simulink model "empirical_cell_twaice_balancing"  (R2024b)
settings: Solver=FixedStepAuto  StartTime=0.0  StopTime=inf  FixedStep=1  RelTol=1e-3
values from neighbouring files (symbols this model uses):
  act = 1    [RunMe_TWAICE_Cell_Model_Farasis_P75_75Ah_v8_1_3.m]
  lic_no = fin_convert(Prod_lic)    [RunMe_TWAICE_Cell_Model_Farasis_P75_75Ah_v8_1_3.m]
  Ts = 1    [RunMe_TWAICE_Cell_Model_Farasis_P75_75Ah_v8_1_3.m]
undefined symbols (not defined in the file or in its folder): DWORK0, DWORK1, DWORK10, DWORK11, DWORK12, DWORK13, DWORK14, DWORK15, DWORK16, DWORK17, DWORK18, DWORK19, DWORK2, DWORK20, DWORK22, DWORK23, DWORK24, DWORK25, DWORK26, DWORK27, DWORK28, DWORK29, DWORK3, DWORK30, DWORK31, DWORK32, DWORK33, DWORK34, DWORK35, DWORK36, DWORK4, DWORK5, DWORK6, DWORK7, DWORK8, DWORK9, SOHc_init, SOHr_init
libraries: fl_lib x73, nesl_utility x32, ee_lib x8
(part 2 of 4)

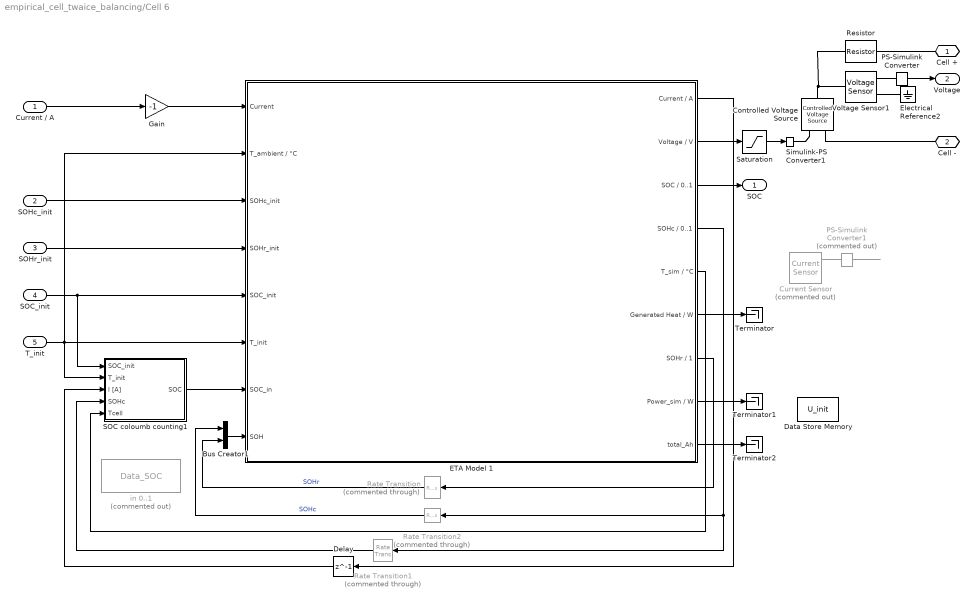
== system empirical_cell_twaice_balancing/Cell 6 ==
  "Current / A " : Inport  OutDataTypeStr=double  PortDimensions=1
  SOHc_init : Inport  Port=2
  SOHr_init : Inport  Port=3
  SOC_init : Inport  Port=4
  T_init : Inport  Port=5
  Bus Creator1 : BusCreator  Inputs=2
  Controlled Voltage Source : fl_lib/Electrical/Electrical Sources/Controlled Voltage Source
  Current Sensor : fl_lib/Electrical/Electrical Sensors/Current Sensor  Commented=on
  Data Store Memory : DataStoreMemory  DataStoreName=U_init  WriteAfterWriteMsg=warning  ShowAdditionalParam=off
  Delay : Delay  DelayLength=1
  ETA Model 1 : Subsystem  mask{sfcnParam1=Ts, sfcnParam2=act, sfcnParam3=lic_no}
      mask prompts: sfcnParam1 "Ts:"; sfcnParam2 "act:"; sfcnParam3 "lic_no:"
      mask help: Simulink:masks:GenSFuncDesc_MD
      mask Help: eval('feval(''rtwprivate'',''rtwhelpview'',''rtw_sfcn_block'')');
  Electrical Reference2 : fl_lib/Electrical/Electrical Elements/Electrical Reference
  Gain : Gain  Gain=-1
  PS-Simulink Converter : nesl_utility/PS-Simulink Converter  PhysicalDomain=network_engine_domain  SubClassName=ps_output  LeftPortType=input  RightPortType=output  PseudoPeriodic=off  Frequencies=[]  VectorFormat=inherit  Unit=inherit  AffineConversion=on
  PS-Simulink Converter1 : nesl_utility/PS-Simulink Converter  Commented=on  PhysicalDomain=network_engine_domain  SubClassName=ps_output  LeftPortType=input  RightPortType=output  PseudoPeriodic=off  Frequencies=[]  VectorFormat=inherit  Unit=inherit  AffineConversion=on
  Rate Transition : RateTransition  Commented=through  InitialCondition=SOHr_init
  Rate Transition1 : RateTransition  Commented=through  InitialCondition=SOHc_init
  Rate Transition2 : RateTransition  Commented=through  InitialCondition=SOHc_init
  Resistor : fl_lib/Electrical/Electrical Elements/Resistor  R=1 mOhm  i_specify=off  i_priority=None  i=0 A  i_nominal_specify=off  i_nominal_value=1  i_nominal_unit=A  v_specify=off  v_priority=None  v=0 V  v_nominal_specify=off  v_nominal_value=1  v_nominal_unit=V
  SOC coloumb counting1 : Subsystem  mask{sfcnParam1=Ts}
      mask prompts: sfcnParam1 "Ts:"
      mask help: Simulink:masks:GenSFuncDesc_MD
      mask Help: eval('feval(''rtwprivate'',''rtwhelpview'',''rtw_sfcn_block'')');
  Saturation : Saturate  UpperLimit=4.15  LowerLimit=2.8
  Simulink-PS Converter1 : nesl_utility/Simulink-PS Converter  PhysicalDomain=network_engine_domain  SubClassName=ps_input  LeftPortType=input  RightPortType=output  PseudoPeriodic=off  Frequencies=[]  NoiseDistribution=none  NoiseParameters=[]  Unit=1  AffineConversion=on  FilteringAndDerivatives=provide  SimscapeFilterOrder=1  InputFilterTimeConstant=0.001  UdotUserProvided=0
  Terminator : Terminator
  Terminator1 : Terminator
  Terminator2 : Terminator
  Voltage Sensor1 : fl_lib/Electrical/Electrical Sensors/Voltage Sensor
  in 0..1 : FromWorkspace  Commented=on  VariableName=Data_SOC  SampleTime=Ts  OutputAfterFinalValue=Setting to zero
  Cell + : PMIOPort  Side=Right
  Cell - : PMIOPort  Port=2  Side=Right
  SOC : Outport
  Voltage : Outport  Port=2
  wires:
  Rate Transition/1 -> Bus Creator1/2  "SOHr"
  T_init/1 -> ETA Model 1/2(T_ambient / °C), SOC coloumb counting1/2(T_init), ETA Model 1/6(T_init)
  ETA Model 1/4(SOHc / 0..1) -> Rate Transition2/1, Rate Transition1/1
  SOC_init/1 -> SOC coloumb counting1/1(SOC_init), ETA Model 1/5(SOC_init)
  Rate Transition1/1 -> SOC coloumb counting1/4(SOHc)
  SOHc_init/1 -> ETA Model 1/3(SOHc_init)
  ETA Model 1/9(total_Ah) -> Terminator2/1
  ETA Model 1/7(SOHr / 1) -> Rate Transition/1
  ETA Model 1/1(Current / A) -> Delay/1
  ETA Model 1/5(T_sim / °C) -> SOC coloumb counting1/5(Tcell)
  SOC coloumb counting1/1(SOC) -> ETA Model 1/7(SOC_in)
  ETA Model 1/8(Power_sim / W) -> Terminator1/1
  Delay/1 -> SOC coloumb counting1/3(I [A])
  Bus Creator1/1 -> ETA Model 1/8(SOH)
  Rate Transition2/1 -> Bus Creator1/1  "SOHc"
  "Current / A "/1 -> Gain/1
  SOHr_init/1 -> ETA Model 1/4(SOHr_init)
  ETA Model 1/6(Generated Heat / W) -> Terminator/1
  Gain/1 -> ETA Model 1/1("Current ")
  ETA Model 1/3(SOC / 0..1) -> SOC/1
  PS-Simulink Converter/1 -> Voltage/1
  ETA Model 1/2(Voltage / V) -> Saturation/1
  PS-Simulink Converter1/1 -> ?
  Saturation/1 -> Simulink-PS Converter1/1
  connections:
  Cell +/RConn1 -- Resistor/RConn1
  Electrical Reference2/LConn1 -- Voltage Sensor1/RConn2
  PS-Simulink Converter/LConn1 -- Voltage Sensor1/RConn1
  Current Sensor/RConn1 -- PS-Simulink Converter1/LConn1
  Controlled Voltage Source/RConn2 -- Cell -/RConn1
  Simulink-PS Converter1/RConn1 -- Controlled Voltage Source/RConn1
  Voltage Sensor1/LConn1 -- Resistor/LConn1 -- Controlled Voltage Source/LConn1

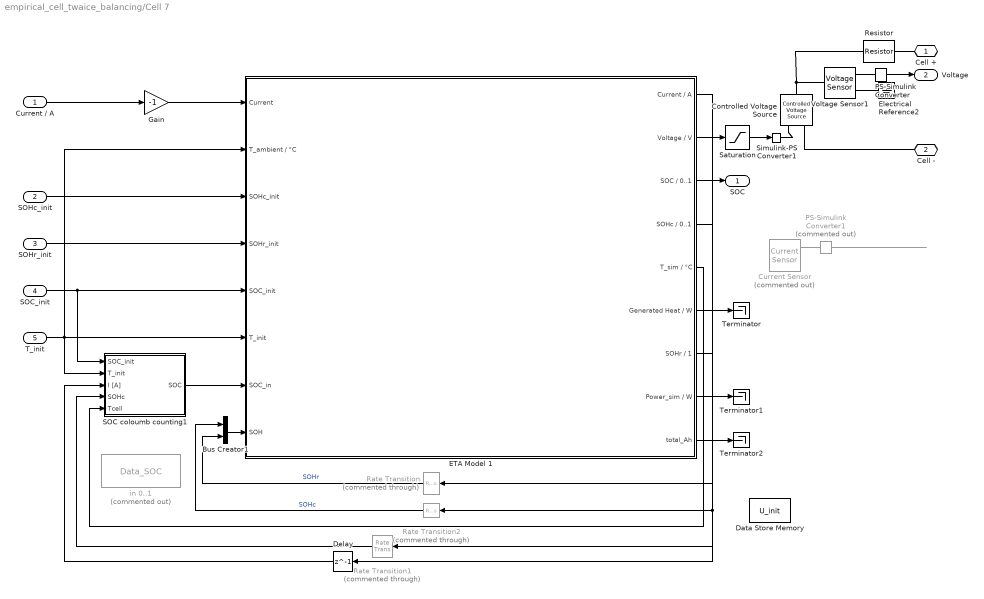
== system empirical_cell_twaice_balancing/Cell 7 ==
  "Current / A " : Inport  OutDataTypeStr=double  PortDimensions=1
  SOHc_init : Inport  Port=2
  SOHr_init : Inport  Port=3
  SOC_init : Inport  Port=4
  T_init : Inport  Port=5
  Bus Creator1 : BusCreator  Inputs=2
  Controlled Voltage Source : fl_lib/Electrical/Electrical Sources/Controlled Voltage Source
  Current Sensor : fl_lib/Electrical/Electrical Sensors/Current Sensor  Commented=on
  Data Store Memory : DataStoreMemory  DataStoreName=U_init  WriteAfterWriteMsg=warning  ShowAdditionalParam=off
  Delay : Delay  DelayLength=1
  ETA Model 1 : Subsystem  mask{sfcnParam1=Ts, sfcnParam2=act, sfcnParam3=lic_no}
      mask prompts: sfcnParam1 "Ts:"; sfcnParam2 "act:"; sfcnParam3 "lic_no:"
      mask help: Simulink:masks:GenSFuncDesc_MD
      mask Help: eval('feval(''rtwprivate'',''rtwhelpview'',''rtw_sfcn_block'')');
  Electrical Reference2 : fl_lib/Electrical/Electrical Elements/Electrical Reference
  Gain : Gain  Gain=-1
  PS-Simulink Converter : nesl_utility/PS-Simulink Converter  PhysicalDomain=network_engine_domain  SubClassName=ps_output  LeftPortType=input  RightPortType=output  PseudoPeriodic=off  Frequencies=[]  VectorFormat=inherit  Unit=inherit  AffineConversion=on
  PS-Simulink Converter1 : nesl_utility/PS-Simulink Converter  Commented=on  PhysicalDomain=network_engine_domain  SubClassName=ps_output  LeftPortType=input  RightPortType=output  PseudoPeriodic=off  Frequencies=[]  VectorFormat=inherit  Unit=inherit  AffineConversion=on
  Rate Transition : RateTransition  Commented=through  InitialCondition=SOHr_init
  Rate Transition1 : RateTransition  Commented=through  InitialCondition=SOHc_init
  Rate Transition2 : RateTransition  Commented=through  InitialCondition=SOHc_init
  Resistor : fl_lib/Electrical/Electrical Elements/Resistor  R=1 mOhm  i_specify=off  i_priority=None  i=0 A  i_nominal_specify=off  i_nominal_value=1  i_nominal_unit=A  v_specify=off  v_priority=None  v=0 V  v_nominal_specify=off  v_nominal_value=1  v_nominal_unit=V
  SOC coloumb counting1 : Subsystem  mask{sfcnParam1=Ts}
      mask prompts: sfcnParam1 "Ts:"
      mask help: Simulink:masks:GenSFuncDesc_MD
      mask Help: eval('feval(''rtwprivate'',''rtwhelpview'',''rtw_sfcn_block'')');
  Saturation : Saturate  UpperLimit=4.15  LowerLimit=2.8
  Simulink-PS Converter1 : nesl_utility/Simulink-PS Converter  PhysicalDomain=network_engine_domain  SubClassName=ps_input  LeftPortType=input  RightPortType=output  PseudoPeriodic=off  Frequencies=[]  NoiseDistribution=none  NoiseParameters=[]  Unit=1  AffineConversion=on  FilteringAndDerivatives=provide  SimscapeFilterOrder=1  InputFilterTimeConstant=0.001  UdotUserProvided=0
  Terminator : Terminator
  Terminator1 : Terminator
  Terminator2 : Terminator
  Voltage Sensor1 : fl_lib/Electrical/Electrical Sensors/Voltage Sensor
  in 0..1 : FromWorkspace  Commented=on  VariableName=Data_SOC  SampleTime=Ts  OutputAfterFinalValue=Setting to zero
  Cell + : PMIOPort  Side=Right
  Cell - : PMIOPort  Port=2  Side=Right
  SOC : Outport
  Voltage : Outport  Port=2
  wires:
  Rate Transition/1 -> Bus Creator1/2  "SOHr"
  T_init/1 -> ETA Model 1/2(T_ambient / °C), SOC coloumb counting1/2(T_init), ETA Model 1/6(T_init)
  ETA Model 1/4(SOHc / 0..1) -> Rate Transition2/1, Rate Transition1/1
  SOC_init/1 -> SOC coloumb counting1/1(SOC_init), ETA Model 1/5(SOC_init)
  Rate Transition1/1 -> SOC coloumb counting1/4(SOHc)
  SOHc_init/1 -> ETA Model 1/3(SOHc_init)
  ETA Model 1/7(SOHr / 1) -> Rate Transition/1
  ETA Model 1/1(Current / A) -> Delay/1
  ETA Model 1/5(T_sim / °C) -> SOC coloumb counting1/5(Tcell)
  SOC coloumb counting1/1(SOC) -> ETA Model 1/7(SOC_in)
  Delay/1 -> SOC coloumb counting1/3(I [A])
  Bus Creator1/1 -> ETA Model 1/8(SOH)
  Rate Transition2/1 -> Bus Creator1/1  "SOHc"
  SOHr_init/1 -> ETA Model 1/4(SOHr_init)
  ETA Model 1/6(Generated Heat / W) -> Terminator/1
  Gain/1 -> ETA Model 1/1("Current ")
  ETA Model 1/8(Power_sim / W) -> Terminator1/1
  ETA Model 1/3(SOC / 0..1) -> SOC/1
  PS-Simulink Converter/1 -> Voltage/1
  "Current / A "/1 -> Gain/1
  ETA Model 1/2(Voltage / V) -> Saturation/1
  ETA Model 1/9(total_Ah) -> Terminator2/1
  PS-Simulink Converter1/1 -> ?
  Saturation/1 -> Simulink-PS Converter1/1
  connections:
  PS-Simulink Converter/LConn1 -- Voltage Sensor1/RConn1
  Simulink-PS Converter1/RConn1 -- Controlled Voltage Source/RConn1
  Voltage Sensor1/LConn1 -- Resistor/LConn1 -- Controlled Voltage Source/LConn1
  Controlled Voltage Source/RConn2 -- Cell -/RConn1
  Electrical Reference2/LConn1 -- Voltage Sensor1/RConn2
  Current Sensor/RConn1 -- PS-Simulink Converter1/LConn1
  Cell +/RConn1 -- Resistor/RConn1

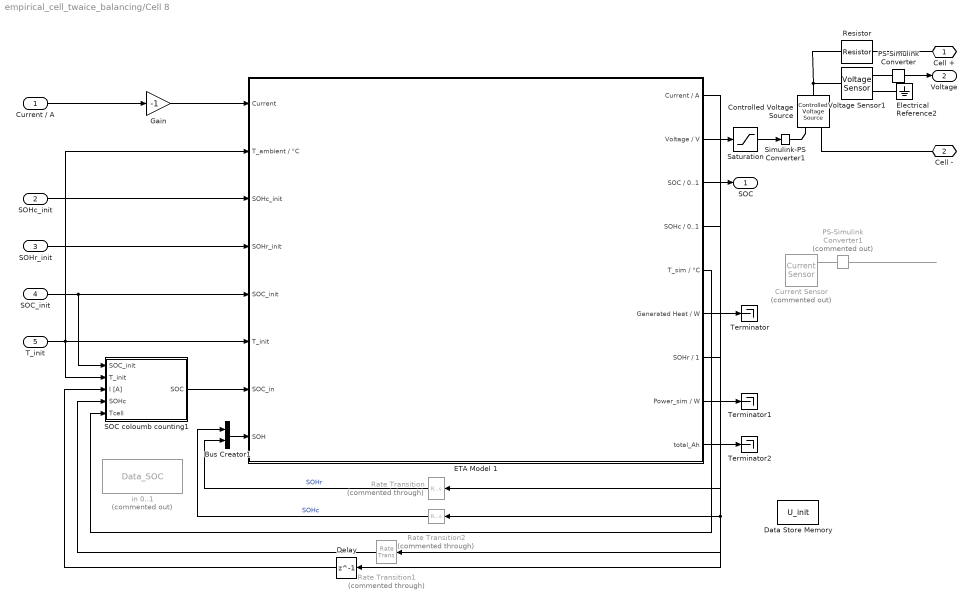
== system empirical_cell_twaice_balancing/Cell 8 ==
  "Current / A " : Inport  OutDataTypeStr=double  PortDimensions=1
  SOHc_init : Inport  Port=2
  SOHr_init : Inport  Port=3
  SOC_init : Inport  Port=4
  T_init : Inport  Port=5
  Bus Creator1 : BusCreator  Inputs=2
  Controlled Voltage Source : fl_lib/Electrical/Electrical Sources/Controlled Voltage Source
  Current Sensor : fl_lib/Electrical/Electrical Sensors/Current Sensor  Commented=on
  Data Store Memory : DataStoreMemory  DataStoreName=U_init  WriteAfterWriteMsg=warning  ShowAdditionalParam=off
  Delay : Delay  DelayLength=1
  ETA Model 1 : Subsystem  mask{sfcnParam1=Ts, sfcnParam2=act, sfcnParam3=lic_no}
      mask prompts: sfcnParam1 "Ts:"; sfcnParam2 "act:"; sfcnParam3 "lic_no:"
      mask help: Simulink:masks:GenSFuncDesc_MD
      mask Help: eval('feval(''rtwprivate'',''rtwhelpview'',''rtw_sfcn_block'')');
  Electrical Reference2 : fl_lib/Electrical/Electrical Elements/Electrical Reference
  Gain : Gain  Gain=-1
  PS-Simulink Converter : nesl_utility/PS-Simulink Converter  PhysicalDomain=network_engine_domain  SubClassName=ps_output  LeftPortType=input  RightPortType=output  PseudoPeriodic=off  Frequencies=[]  VectorFormat=inherit  Unit=inherit  AffineConversion=on
  PS-Simulink Converter1 : nesl_utility/PS-Simulink Converter  Commented=on  PhysicalDomain=network_engine_domain  SubClassName=ps_output  LeftPortType=input  RightPortType=output  PseudoPeriodic=off  Frequencies=[]  VectorFormat=inherit  Unit=inherit  AffineConversion=on
  Rate Transition : RateTransition  Commented=through  InitialCondition=SOHr_init
  Rate Transition1 : RateTransition  Commented=through  InitialCondition=SOHc_init
  Rate Transition2 : RateTransition  Commented=through  InitialCondition=SOHc_init
  Resistor : fl_lib/Electrical/Electrical Elements/Resistor  R=1 mOhm  i_specify=off  i_priority=None  i=0 A  i_nominal_specify=off  i_nominal_value=1  i_nominal_unit=A  v_specify=off  v_priority=None  v=0 V  v_nominal_specify=off  v_nominal_value=1  v_nominal_unit=V
  SOC coloumb counting1 : Subsystem  mask{sfcnParam1=Ts}
      mask prompts: sfcnParam1 "Ts:"
      mask help: Simulink:masks:GenSFuncDesc_MD
      mask Help: eval('feval(''rtwprivate'',''rtwhelpview'',''rtw_sfcn_block'')');
  Saturation : Saturate  UpperLimit=4.15  LowerLimit=2.8
  Simulink-PS Converter1 : nesl_utility/Simulink-PS Converter  PhysicalDomain=network_engine_domain  SubClassName=ps_input  LeftPortType=input  RightPortType=output  PseudoPeriodic=off  Frequencies=[]  NoiseDistribution=none  NoiseParameters=[]  Unit=1  AffineConversion=on  FilteringAndDerivatives=provide  SimscapeFilterOrder=1  InputFilterTimeConstant=0.001  UdotUserProvided=0
  Terminator : Terminator
  Terminator1 : Terminator
  Terminator2 : Terminator
  Voltage Sensor1 : fl_lib/Electrical/Electrical Sensors/Voltage Sensor
  in 0..1 : FromWorkspace  Commented=on  VariableName=Data_SOC  SampleTime=Ts  OutputAfterFinalValue=Setting to zero
  Cell + : PMIOPort  Side=Right
  Cell - : PMIOPort  Port=2  Side=Right
  SOC : Outport
  Voltage : Outport  Port=2
  wires:
  Rate Transition/1 -> Bus Creator1/2  "SOHr"
  T_init/1 -> ETA Model 1/2(T_ambient / °C), SOC coloumb counting1/2(T_init), ETA Model 1/6(T_init)
  ETA Model 1/4(SOHc / 0..1) -> Rate Transition2/1, Rate Transition1/1
  SOC_init/1 -> SOC coloumb counting1/1(SOC_init), ETA Model 1/5(SOC_init)
  Rate Transition1/1 -> SOC coloumb counting1/4(SOHc)
  SOHc_init/1 -> ETA Model 1/3(SOHc_init)
  ETA Model 1/7(SOHr / 1) -> Rate Transition/1
  ETA Model 1/1(Current / A) -> Delay/1
  ETA Model 1/5(T_sim / °C) -> SOC coloumb counting1/5(Tcell)
  SOC coloumb counting1/1(SOC) -> ETA Model 1/7(SOC_in)
  Delay/1 -> SOC coloumb counting1/3(I [A])
  Bus Creator1/1 -> ETA Model 1/8(SOH)
  Rate Transition2/1 -> Bus Creator1/1  "SOHc"
  SOHr_init/1 -> ETA Model 1/4(SOHr_init)
  Gain/1 -> ETA Model 1/1("Current ")
  PS-Simulink Converter/1 -> Voltage/1
  "Current / A "/1 -> Gain/1
  ETA Model 1/9(total_Ah) -> Terminator2/1
  ETA Model 1/3(SOC / 0..1) -> SOC/1
  ETA Model 1/2(Voltage / V) -> Saturation/1
  ETA Model 1/8(Power_sim / W) -> Terminator1/1
  ETA Model 1/6(Generated Heat / W) -> Terminator/1
  PS-Simulink Converter1/1 -> ?
  Saturation/1 -> Simulink-PS Converter1/1
  connections:
  Electrical Reference2/LConn1 -- Voltage Sensor1/RConn2
  Voltage Sensor1/LConn1 -- Resistor/LConn1 -- Controlled Voltage Source/LConn1
  Simulink-PS Converter1/RConn1 -- Controlled Voltage Source/RConn1
  Controlled Voltage Source/RConn2 -- Cell -/RConn1
  PS-Simulink Converter/LConn1 -- Voltage Sensor1/RConn1
  PS-Simulink Converter1/LConn1 -- Current Sensor/RConn1
  Cell +/RConn1 -- Resistor/RConn1

== system empirical_cell_twaice_balancing/Cell 1/ETA Model 1 ==
  "Current " : Inport  OutDataTypeStr=double  PortDimensions=1
  T_ambient / °C : Inport  Port=2  OutDataTypeStr=double  PortDimensions=1
  SOHc_init : Inport  Port=3
  SOHr_init : Inport  Port=4
  SOC_init : Inport  Port=5
  T_init : Inport  Port=6
  SOC_in : Inport  Port=7
  SOH : Inport  Port=8
  ETA Model _sfcn : S-Function  FunctionName=ETA_sf  Parameters=sfcnParam1, sfcnParam2, sfcnParam3  SFunctionModules=""  SFunctionDeploymentMode=off  EnableBusSupport=off  SFcnStateName=DWORK0,DWORK1,DWORK2,DWORK3,DWORK4,DWORK5,DWORK6,DWORK7,DWORK8,DWORK9,DWORK10,DWORK11,DWORK12,DWORK13,DWORK14,DWORK15,DWORK16,DWORK17,DWORK18,DWORK19,DWORK20,DWORK22,DWORK23,DWORK24,DWORK25,DWORK26,DWORK27,DWORK28,DWORK29,DWORK30,DWORK31,DWORK32,DWORK33,DWORK34,DWORK35,DWORK36  mask{rtw_sf_name=ETA_sf, showVar=off, sfcnParam1=sfcnParam1, sfcnParam2=sfcnParam2, sfcnParam3=sfcnParam3}
      mask prompts: rtw_sf_name "Simulink:masks:GenSFuncName_MP"; showVar "Simulink:masks:GenSFuncShowModuleList_MP"; sfcnParam1 "Ts:"; sfcnParam2 "act:"; sfcnParam3 "lic_no:"
      mask help: Simulink:masks:GenSFuncDesc_MD
      mask init:
      | displist = '';
      | if ~strcmp(get_param(gcb, 'FunctionName'), rtw_sf_name);
      |   set_param(gcb, 'FunctionName', rtw_sf_name);
      | end
      | % Check if we are generating code
      | rtw_mode = false;
      | if strcmpi(get_param(bdroot(gcb),'SimulationStatus'),'Initializing')
      | 	rtw_mode = strcmpi(get_param(bdroot(gcb),'BuildingRTWCode'),'on') && ...
      | 		~strcmpi(get_param(bdroot(gcb),'TargetStyle'),'SimulationTarget');
      | end
      | if showVar || rtw_mode
      | 	if exist('rtwsfunc') == 2 | exist('rtwsfunc') == 6
      | 		tmplist = rtwsfunc(rtw_sf_name,gcb);
      | 		tmplist = DAStudio.message('Simulink:masks:GenSFuncListOfModules_IC', tmplist);
      | 	elseif showVar
      | 		tmplist1 = DAStudio.message('Simulink:masks:GenSFuncListOfModules_IC', '');
      |         tmplist2 = DAStudio.message('Simulink:masks:GenSFuncNotLicensed_IC');
      |         tmplist = [tmplist1 tmplist2];
      |  	end
      | end
      | if showVar
      |   displist = tmplist;
      | end
      settings: SFcnIsStateOwnerBlock=on
      settings: CopyFcn=|
      | if ~strcmp(get_param(gcb,'Linkstatus'),'none') && ...
      | ~strcmp(get_param(gcb,'Linkstatus'),'implicit')
      |   set_param(gcb,'LinkStatus','none');
      | end
      mask Help: eval('feval(''rtwprivate'',''rtwhelpview'',''rtw_sfcn_block'')');
      mask Display:
      | port_label('input',1,'Current ');
      | port_label('input',2,'T_ambient / °C');
      | port_label('input',3,'htc_in');
      | port_label('input',4,'Pcool_in');
      | port_label('input',5,'SOHc_init');
      | port_label('input',6,'SOHr_init');
      | port_label('input',7,'SOC_init');
      | port_label('input',8,'T_init');
      | port_label('input',9,'SOC_in');
      | port_label('input',10,'SOHc');
      | port_label('input',11,'SOHr');
      | port_label('output',1,'Current / A');
      | port_label('output',2,'Voltage / V');
      | port_label('output',3,'SOC / 0..1');
      | port_label('output',4,'SOHc / 0..1');
      | port_label('output',5,'T_sim / °C');
      | port_label('output',6,'Generated Heat / W');
      | port_label('output',7,'SOHr / 1');
      | port_label('output',8,'Power_sim / W');
      | port_label('output',9,'total_Ah');
  __InputSSForSFun__ : Subsystem
  __OutputSSForSFun__ : Subsystem
  Current / A : Outport  OutDataTypeStr=double  PortDimensions=1
  Voltage / V : Outport  Port=2  OutDataTypeStr=double  PortDimensions=1
  SOC / 0..1 : Outport  Port=3  OutDataTypeStr=double  PortDimensions=1
  SOHc / 0..1 : Outport  Port=4  OutDataTypeStr=double  PortDimensions=1
  T_sim / °C : Outport  Port=5  OutDataTypeStr=double  PortDimensions=1
  Generated Heat / W : Outport  Port=6  OutDataTypeStr=double  PortDimensions=1
  SOHr / 1 : Outport  Port=7  OutDataTypeStr=double  PortDimensions=1
  Power_sim / W : Outport  Port=8  OutDataTypeStr=double  PortDimensions=1
  total_Ah : Outport  Port=9
  wires:
  "Current "/1 -> __InputSSForSFun__/1("Current ")
  T_ambient / °C/1 -> __InputSSForSFun__/2(T_ambient / °C)
  SOHc_init/1 -> __InputSSForSFun__/3(SOHc_init)
  SOHr_init/1 -> __InputSSForSFun__/4(SOHr_init)
  SOC_init/1 -> __InputSSForSFun__/5(SOC_init)
  T_init/1 -> __InputSSForSFun__/6(T_init)
  SOC_in/1 -> __InputSSForSFun__/7(SOC_in)
  SOH/1 -> __InputSSForSFun__/8(SOH)
  __InputSSForSFun__/1(__UniqueOutportName__1__) -> ETA Model _sfcn/1
  __InputSSForSFun__/2(__UniqueOutportName__2__) -> ETA Model _sfcn/2
  __InputSSForSFun__/3(__UniqueOutportName__3__) -> ETA Model _sfcn/3
  __InputSSForSFun__/4(__UniqueOutportName__4__) -> ETA Model _sfcn/4
  __InputSSForSFun__/5(__UniqueOutportName__5__) -> ETA Model _sfcn/5
  __InputSSForSFun__/6(__UniqueOutportName__6__) -> ETA Model _sfcn/6
  __InputSSForSFun__/7(__UniqueOutportName__7__) -> ETA Model _sfcn/7
  __InputSSForSFun__/8(__UniqueOutportName__8__) -> ETA Model _sfcn/8
  __InputSSForSFun__/9(__UniqueOutportName__9__) -> ETA Model _sfcn/9
  __InputSSForSFun__/10(__UniqueOutportName__10__) -> ETA Model _sfcn/10
  __InputSSForSFun__/11(__UniqueOutportName__11__) -> ETA Model _sfcn/11
  ETA Model _sfcn/1 -> __OutputSSForSFun__/1(__UniqueInportName__1__)
  ETA Model _sfcn/2 -> __OutputSSForSFun__/2(__UniqueInportName__2__)
  ETA Model _sfcn/3 -> __OutputSSForSFun__/3(__UniqueInportName__3__)
  ETA Model _sfcn/4 -> __OutputSSForSFun__/4(__UniqueInportName__4__)
  ETA Model _sfcn/5 -> __OutputSSForSFun__/5(__UniqueInportName__5__)
  ETA Model _sfcn/6 -> __OutputSSForSFun__/6(__UniqueInportName__6__)
  ETA Model _sfcn/7 -> __OutputSSForSFun__/7(__UniqueInportName__7__)
  ETA Model _sfcn/8 -> __OutputSSForSFun__/8(__UniqueInportName__8__)
  ETA Model _sfcn/9 -> __OutputSSForSFun__/9(__UniqueInportName__9__)
  __OutputSSForSFun__/1(Current / A) -> Current / A/1
  __OutputSSForSFun__/2(Voltage / V) -> Voltage / V/1
  __OutputSSForSFun__/3(SOC / 0..1) -> SOC / 0..1/1
  __OutputSSForSFun__/4(SOHc / 0..1) -> SOHc / 0..1/1
  __OutputSSForSFun__/5(T_sim / °C) -> T_sim / °C/1
  __OutputSSForSFun__/6(Generated Heat / W) -> Generated Heat / W/1
  __OutputSSForSFun__/7(SOHr / 1) -> SOHr / 1/1
  __OutputSSForSFun__/8(Power_sim / W) -> Power_sim / W/1
  __OutputSSForSFun__/9(total_Ah) -> total_Ah/1

== system empirical_cell_twaice_balancing/Cell 1/SOC coloumb counting1 ==
  SOC_init : Inport
  T_init : Inport  Port=2
  I [A] : Inport  Port=3
  SOHc : Inport  Port=4
  Tcell : Inport  Port=5
  SOC coloumb counting_sfcn : S-Function  FunctionName=SOC_sf  Parameters=sfcnParam1  SFunctionModules=""  SFunctionDeploymentMode=off  EnableBusSupport=off  SFcnStateName=DWORK0,DWORK1  mask{rtw_sf_name=SOC_sf, showVar=off, sfcnParam1=sfcnParam1}
      mask prompts: rtw_sf_name "Simulink:masks:GenSFuncName_MP"; showVar "Simulink:masks:GenSFuncShowModuleList_MP"; sfcnParam1 "Ts:"
      mask help: Simulink:masks:GenSFuncDesc_MD
      mask init: same as empirical_cell_twaice_balancing/Cell 1/ETA Model 1/ETA Model _sfcn
      settings: SFcnIsStateOwnerBlock=on
      settings: CopyFcn=|
      | if ~strcmp(get_param(gcb,'Linkstatus'),'none') && ...
      | ~strcmp(get_param(gcb,'Linkstatus'),'implicit')
      |   set_param(gcb,'LinkStatus','none');
      | end
      mask Help: eval('feval(''rtwprivate'',''rtwhelpview'',''rtw_sfcn_block'')');
      mask Display:
      | port_label('input',1,'SOC_init');
      | port_label('input',2,'T_init');
      | port_label('input',3,'I [A]');
      | port_label('input',4,'SOHc');
      | port_label('input',5,'Tcell');
      | port_label('output',1,'SOC');
  __InputSSForSFun__ : Subsystem
  __OutputSSForSFun__ : Subsystem
  SOC : Outport  VectorParamsAs1DForOutWhenUnconnected=off
  wires:
  SOC_init/1 -> __InputSSForSFun__/1(SOC_init)
  T_init/1 -> __InputSSForSFun__/2(T_init)
  I [A]/1 -> __InputSSForSFun__/3(I [A])
  SOHc/1 -> __InputSSForSFun__/4(SOHc)
  Tcell/1 -> __InputSSForSFun__/5(Tcell)
  __InputSSForSFun__/1(__UniqueOutportName__1__) -> SOC coloumb counting_sfcn/1
  __InputSSForSFun__/2(__UniqueOutportName__2__) -> SOC coloumb counting_sfcn/2
  __InputSSForSFun__/3(__UniqueOutportName__3__) -> SOC coloumb counting_sfcn/3
  __InputSSForSFun__/4(__UniqueOutportName__4__) -> SOC coloumb counting_sfcn/4
  __InputSSForSFun__/5(__UniqueOutportName__5__) -> SOC coloumb counting_sfcn/5
  SOC coloumb counting_sfcn/1 -> __OutputSSForSFun__/1(__UniqueInportName__1__)
  __OutputSSForSFun__/1(SOC) -> SOC/1

== system empirical_cell_twaice_balancing/Cell 2/ETA Model 1 ==
  "Current " : Inport  OutDataTypeStr=double  PortDimensions=1
  T_ambient / °C : Inport  Port=2  OutDataTypeStr=double  PortDimensions=1
  SOHc_init : Inport  Port=3
  SOHr_init : Inport  Port=4
  SOC_init : Inport  Port=5
  T_init : Inport  Port=6
  SOC_in : Inport  Port=7
  SOH : Inport  Port=8
  ETA Model _sfcn : S-Function  FunctionName=ETA_sf  Parameters=sfcnParam1, sfcnParam2, sfcnParam3  SFunctionModules=""  SFunctionDeploymentMode=off  EnableBusSupport=off  SFcnStateName=DWORK0,DWORK1,DWORK2,DWORK3,DWORK4,DWORK5,DWORK6,DWORK7,DWORK8,DWORK9,DWORK10,DWORK11,DWORK12,DWORK13,DWORK14,DWORK15,DWORK16,DWORK17,DWORK18,DWORK19,DWORK20,DWORK22,DWORK23,DWORK24,DWORK25,DWORK26,DWORK27,DWORK28,DWORK29,DWORK30,DWORK31,DWORK32,DWORK33,DWORK34,DWORK35,DWORK36  mask{rtw_sf_name=ETA_sf, showVar=off, sfcnParam1=sfcnParam1, sfcnParam2=sfcnParam2, sfcnParam3=sfcnParam3}
      mask prompts: rtw_sf_name "Simulink:masks:GenSFuncName_MP"; showVar "Simulink:masks:GenSFuncShowModuleList_MP"; sfcnParam1 "Ts:"; sfcnParam2 "act:"; sfcnParam3 "lic_no:"
      mask help: Simulink:masks:GenSFuncDesc_MD
      mask init: same as empirical_cell_twaice_balancing/Cell 1/ETA Model 1/ETA Model _sfcn
      settings: SFcnIsStateOwnerBlock=on
      settings: CopyFcn=|
      | if ~strcmp(get_param(gcb,'Linkstatus'),'none') && ...
      | ~strcmp(get_param(gcb,'Linkstatus'),'implicit')
      |   set_param(gcb,'LinkStatus','none');
      | end
      mask Help: eval('feval(''rtwprivate'',''rtwhelpview'',''rtw_sfcn_block'')');
      mask Display:
      | port_label('input',1,'Current ');
      | port_label('input',2,'T_ambient / °C');
      | port_label('input',3,'htc_in');
      | port_label('input',4,'Pcool_in');
      | port_label('input',5,'SOHc_init');
      | port_label('input',6,'SOHr_init');
      | port_label('input',7,'SOC_init');
      | port_label('input',8,'T_init');
      | port_label('input',9,'SOC_in');
      | port_label('input',10,'SOHc');
      | port_label('input',11,'SOHr');
      | port_label('output',1,'Current / A');
      | port_label('output',2,'Voltage / V');
      | port_label('output',3,'SOC / 0..1');
      | port_label('output',4,'SOHc / 0..1');
      | port_label('output',5,'T_sim / °C');
      | port_label('output',6,'Generated Heat / W');
      | port_label('output',7,'SOHr / 1');
      | port_label('output',8,'Power_sim / W');
      | port_label('output',9,'total_Ah');
  __InputSSForSFun__ : Subsystem
  __OutputSSForSFun__ : Subsystem
  Current / A : Outport  OutDataTypeStr=double  PortDimensions=1
  Voltage / V : Outport  Port=2  OutDataTypeStr=double  PortDimensions=1
  SOC / 0..1 : Outport  Port=3  OutDataTypeStr=double  PortDimensions=1
  SOHc / 0..1 : Outport  Port=4  OutDataTypeStr=double  PortDimensions=1
  T_sim / °C : Outport  Port=5  OutDataTypeStr=double  PortDimensions=1
  Generated Heat / W : Outport  Port=6  OutDataTypeStr=double  PortDimensions=1
  SOHr / 1 : Outport  Port=7  OutDataTypeStr=double  PortDimensions=1
  Power_sim / W : Outport  Port=8  OutDataTypeStr=double  PortDimensions=1
  total_Ah : Outport  Port=9
  wires:
  "Current "/1 -> __InputSSForSFun__/1("Current ")
  T_ambient / °C/1 -> __InputSSForSFun__/2(T_ambient / °C)
  SOHc_init/1 -> __InputSSForSFun__/3(SOHc_init)
  SOHr_init/1 -> __InputSSForSFun__/4(SOHr_init)
  SOC_init/1 -> __InputSSForSFun__/5(SOC_init)
  T_init/1 -> __InputSSForSFun__/6(T_init)
  SOC_in/1 -> __InputSSForSFun__/7(SOC_in)
  SOH/1 -> __InputSSForSFun__/8(SOH)
  __InputSSForSFun__/1(__UniqueOutportName__1__) -> ETA Model _sfcn/1
  __InputSSForSFun__/2(__UniqueOutportName__2__) -> ETA Model _sfcn/2
  __InputSSForSFun__/3(__UniqueOutportName__3__) -> ETA Model _sfcn/3
  __InputSSForSFun__/4(__UniqueOutportName__4__) -> ETA Model _sfcn/4
  __InputSSForSFun__/5(__UniqueOutportName__5__) -> ETA Model _sfcn/5
  __InputSSForSFun__/6(__UniqueOutportName__6__) -> ETA Model _sfcn/6
  __InputSSForSFun__/7(__UniqueOutportName__7__) -> ETA Model _sfcn/7
  __InputSSForSFun__/8(__UniqueOutportName__8__) -> ETA Model _sfcn/8
  __InputSSForSFun__/9(__UniqueOutportName__9__) -> ETA Model _sfcn/9
  __InputSSForSFun__/10(__UniqueOutportName__10__) -> ETA Model _sfcn/10
  __InputSSForSFun__/11(__UniqueOutportName__11__) -> ETA Model _sfcn/11
  ETA Model _sfcn/1 -> __OutputSSForSFun__/1(__UniqueInportName__1__)
  ETA Model _sfcn/2 -> __OutputSSForSFun__/2(__UniqueInportName__2__)
  ETA Model _sfcn/3 -> __OutputSSForSFun__/3(__UniqueInportName__3__)
  ETA Model _sfcn/4 -> __OutputSSForSFun__/4(__UniqueInportName__4__)
  ETA Model _sfcn/5 -> __OutputSSForSFun__/5(__UniqueInportName__5__)
  ETA Model _sfcn/6 -> __OutputSSForSFun__/6(__UniqueInportName__6__)
  ETA Model _sfcn/7 -> __OutputSSForSFun__/7(__UniqueInportName__7__)
  ETA Model _sfcn/8 -> __OutputSSForSFun__/8(__UniqueInportName__8__)
  ETA Model _sfcn/9 -> __OutputSSForSFun__/9(__UniqueInportName__9__)
  __OutputSSForSFun__/1(Current / A) -> Current / A/1
  __OutputSSForSFun__/2(Voltage / V) -> Voltage / V/1
  __OutputSSForSFun__/3(SOC / 0..1) -> SOC / 0..1/1
  __OutputSSForSFun__/4(SOHc / 0..1) -> SOHc / 0..1/1
  __OutputSSForSFun__/5(T_sim / °C) -> T_sim / °C/1
  __OutputSSForSFun__/6(Generated Heat / W) -> Generated Heat / W/1
  __OutputSSForSFun__/7(SOHr / 1) -> SOHr / 1/1
  __OutputSSForSFun__/8(Power_sim / W) -> Power_sim / W/1
  __OutputSSForSFun__/9(total_Ah) -> total_Ah/1

== system empirical_cell_twaice_balancing/Cell 2/SOC coloumb counting1 ==
  SOC_init : Inport
  T_init : Inport  Port=2
  I [A] : Inport  Port=3
  SOHc : Inport  Port=4
  Tcell : Inport  Port=5
  SOC coloumb counting_sfcn : S-Function  FunctionName=SOC_sf  Parameters=sfcnParam1  SFunctionModules=""  SFunctionDeploymentMode=off  EnableBusSupport=off  SFcnStateName=DWORK0,DWORK1  mask{rtw_sf_name=SOC_sf, showVar=off, sfcnParam1=sfcnParam1}
      mask prompts: rtw_sf_name "Simulink:masks:GenSFuncName_MP"; showVar "Simulink:masks:GenSFuncShowModuleList_MP"; sfcnParam1 "Ts:"
      mask help: Simulink:masks:GenSFuncDesc_MD
      mask init: same as empirical_cell_twaice_balancing/Cell 1/ETA Model 1/ETA Model _sfcn
      settings: SFcnIsStateOwnerBlock=on
      settings: CopyFcn=|
      | if ~strcmp(get_param(gcb,'Linkstatus'),'none') && ...
      | ~strcmp(get_param(gcb,'Linkstatus'),'implicit')
      |   set_param(gcb,'LinkStatus','none');
      | end
      mask Help: eval('feval(''rtwprivate'',''rtwhelpview'',''rtw_sfcn_block'')');
      mask Display:
      | port_label('input',1,'SOC_init');
      | port_label('input',2,'T_init');
      | port_label('input',3,'I [A]');
      | port_label('input',4,'SOHc');
      | port_label('input',5,'Tcell');
      | port_label('output',1,'SOC');
  __InputSSForSFun__ : Subsystem
  __OutputSSForSFun__ : Subsystem
  SOC : Outport  VectorParamsAs1DForOutWhenUnconnected=off
  wires:
  SOC_init/1 -> __InputSSForSFun__/1(SOC_init)
  T_init/1 -> __InputSSForSFun__/2(T_init)
  I [A]/1 -> __InputSSForSFun__/3(I [A])
  SOHc/1 -> __InputSSForSFun__/4(SOHc)
  Tcell/1 -> __InputSSForSFun__/5(Tcell)
  __InputSSForSFun__/1(__UniqueOutportName__1__) -> SOC coloumb counting_sfcn/1
  __InputSSForSFun__/2(__UniqueOutportName__2__) -> SOC coloumb counting_sfcn/2
  __InputSSForSFun__/3(__UniqueOutportName__3__) -> SOC coloumb counting_sfcn/3
  __InputSSForSFun__/4(__UniqueOutportName__4__) -> SOC coloumb counting_sfcn/4
  __InputSSForSFun__/5(__UniqueOutportName__5__) -> SOC coloumb counting_sfcn/5
  SOC coloumb counting_sfcn/1 -> __OutputSSForSFun__/1(__UniqueInportName__1__)
  __OutputSSForSFun__/1(SOC) -> SOC/1

== system empirical_cell_twaice_balancing/Cell 3/ETA Model 1 ==
  "Current " : Inport  OutDataTypeStr=double  PortDimensions=1
  T_ambient / °C : Inport  Port=2  OutDataTypeStr=double  PortDimensions=1
  SOHc_init : Inport  Port=3
  SOHr_init : Inport  Port=4
  SOC_init : Inport  Port=5
  T_init : Inport  Port=6
  SOC_in : Inport  Port=7
  SOH : Inport  Port=8
  ETA Model _sfcn : S-Function  FunctionName=ETA_sf  Parameters=sfcnParam1, sfcnParam2, sfcnParam3  SFunctionModules=""  SFunctionDeploymentMode=off  EnableBusSupport=off  SFcnStateName=DWORK0,DWORK1,DWORK2,DWORK3,DWORK4,DWORK5,DWORK6,DWORK7,DWORK8,DWORK9,DWORK10,DWORK11,DWORK12,DWORK13,DWORK14,DWORK15,DWORK16,DWORK17,DWORK18,DWORK19,DWORK20,DWORK22,DWORK23,DWORK24,DWORK25,DWORK26,DWORK27,DWORK28,DWORK29,DWORK30,DWORK31,DWORK32,DWORK33,DWORK34,DWORK35,DWORK36  mask{rtw_sf_name=ETA_sf, showVar=off, sfcnParam1=sfcnParam1, sfcnParam2=sfcnParam2, sfcnParam3=sfcnParam3}
      mask prompts: rtw_sf_name "Simulink:masks:GenSFuncName_MP"; showVar "Simulink:masks:GenSFuncShowModuleList_MP"; sfcnParam1 "Ts:"; sfcnParam2 "act:"; sfcnParam3 "lic_no:"
      mask help: Simulink:masks:GenSFuncDesc_MD
      mask init: same as empirical_cell_twaice_balancing/Cell 1/ETA Model 1/ETA Model _sfcn
      settings: SFcnIsStateOwnerBlock=on
      settings: CopyFcn=|
      | if ~strcmp(get_param(gcb,'Linkstatus'),'none') && ...
      | ~strcmp(get_param(gcb,'Linkstatus'),'implicit')
      |   set_param(gcb,'LinkStatus','none');
      | end
      mask Help: eval('feval(''rtwprivate'',''rtwhelpview'',''rtw_sfcn_block'')');
      mask Display:
      | port_label('input',1,'Current ');
      | port_label('input',2,'T_ambient / °C');
      | port_label('input',3,'htc_in');
      | port_label('input',4,'Pcool_in');
      | port_label('input',5,'SOHc_init');
      | port_label('input',6,'SOHr_init');
      | port_label('input',7,'SOC_init');
      | port_label('input',8,'T_init');
      | port_label('input',9,'SOC_in');
      | port_label('input',10,'SOHc');
      | port_label('input',11,'SOHr');
      | port_label('output',1,'Current / A');
      | port_label('output',2,'Voltage / V');
      | port_label('output',3,'SOC / 0..1');
      | port_label('output',4,'SOHc / 0..1');
      | port_label('output',5,'T_sim / °C');
      | port_label('output',6,'Generated Heat / W');
      | port_label('output',7,'SOHr / 1');
      | port_label('output',8,'Power_sim / W');
      | port_label('output',9,'total_Ah');
  __InputSSForSFun__ : Subsystem
  __OutputSSForSFun__ : Subsystem
  Current / A : Outport  OutDataTypeStr=double  PortDimensions=1
  Voltage / V : Outport  Port=2  OutDataTypeStr=double  PortDimensions=1
  SOC / 0..1 : Outport  Port=3  OutDataTypeStr=double  PortDimensions=1
  SOHc / 0..1 : Outport  Port=4  OutDataTypeStr=double  PortDimensions=1
  T_sim / °C : Outport  Port=5  OutDataTypeStr=double  PortDimensions=1
  Generated Heat / W : Outport  Port=6  OutDataTypeStr=double  PortDimensions=1
  SOHr / 1 : Outport  Port=7  OutDataTypeStr=double  PortDimensions=1
  Power_sim / W : Outport  Port=8  OutDataTypeStr=double  PortDimensions=1
  total_Ah : Outport  Port=9
  wires:
  "Current "/1 -> __InputSSForSFun__/1("Current ")
  T_ambient / °C/1 -> __InputSSForSFun__/2(T_ambient / °C)
  SOHc_init/1 -> __InputSSForSFun__/3(SOHc_init)
  SOHr_init/1 -> __InputSSForSFun__/4(SOHr_init)
  SOC_init/1 -> __InputSSForSFun__/5(SOC_init)
  T_init/1 -> __InputSSForSFun__/6(T_init)
  SOC_in/1 -> __InputSSForSFun__/7(SOC_in)
  SOH/1 -> __InputSSForSFun__/8(SOH)
  __InputSSForSFun__/1(__UniqueOutportName__1__) -> ETA Model _sfcn/1
  __InputSSForSFun__/2(__UniqueOutportName__2__) -> ETA Model _sfcn/2
  __InputSSForSFun__/3(__UniqueOutportName__3__) -> ETA Model _sfcn/3
  __InputSSForSFun__/4(__UniqueOutportName__4__) -> ETA Model _sfcn/4
  __InputSSForSFun__/5(__UniqueOutportName__5__) -> ETA Model _sfcn/5
  __InputSSForSFun__/6(__UniqueOutportName__6__) -> ETA Model _sfcn/6
  __InputSSForSFun__/7(__UniqueOutportName__7__) -> ETA Model _sfcn/7
  __InputSSForSFun__/8(__UniqueOutportName__8__) -> ETA Model _sfcn/8
  __InputSSForSFun__/9(__UniqueOutportName__9__) -> ETA Model _sfcn/9
  __InputSSForSFun__/10(__UniqueOutportName__10__) -> ETA Model _sfcn/10
  __InputSSForSFun__/11(__UniqueOutportName__11__) -> ETA Model _sfcn/11
  ETA Model _sfcn/1 -> __OutputSSForSFun__/1(__UniqueInportName__1__)
  ETA Model _sfcn/2 -> __OutputSSForSFun__/2(__UniqueInportName__2__)
  ETA Model _sfcn/3 -> __OutputSSForSFun__/3(__UniqueInportName__3__)
  ETA Model _sfcn/4 -> __OutputSSForSFun__/4(__UniqueInportName__4__)
  ETA Model _sfcn/5 -> __OutputSSForSFun__/5(__UniqueInportName__5__)
  ETA Model _sfcn/6 -> __OutputSSForSFun__/6(__UniqueInportName__6__)
  ETA Model _sfcn/7 -> __OutputSSForSFun__/7(__UniqueInportName__7__)
  ETA Model _sfcn/8 -> __OutputSSForSFun__/8(__UniqueInportName__8__)
  ETA Model _sfcn/9 -> __OutputSSForSFun__/9(__UniqueInportName__9__)
  __OutputSSForSFun__/1(Current / A) -> Current / A/1
  __OutputSSForSFun__/2(Voltage / V) -> Voltage / V/1
  __OutputSSForSFun__/3(SOC / 0..1) -> SOC / 0..1/1
  __OutputSSForSFun__/4(SOHc / 0..1) -> SOHc / 0..1/1
  __OutputSSForSFun__/5(T_sim / °C) -> T_sim / °C/1
  __OutputSSForSFun__/6(Generated Heat / W) -> Generated Heat / W/1
  __OutputSSForSFun__/7(SOHr / 1) -> SOHr / 1/1
  __OutputSSForSFun__/8(Power_sim / W) -> Power_sim / W/1
  __OutputSSForSFun__/9(total_Ah) -> total_Ah/1

== system empirical_cell_twaice_balancing/Cell 3/SOC coloumb counting1 ==
  SOC_init : Inport
  T_init : Inport  Port=2
  I [A] : Inport  Port=3
  SOHc : Inport  Port=4
  Tcell : Inport  Port=5
  SOC coloumb counting_sfcn : S-Function  FunctionName=SOC_sf  Parameters=sfcnParam1  SFunctionModules=""  SFunctionDeploymentMode=off  EnableBusSupport=off  SFcnStateName=DWORK0,DWORK1  mask{rtw_sf_name=SOC_sf, showVar=off, sfcnParam1=sfcnParam1}
      mask prompts: rtw_sf_name "Simulink:masks:GenSFuncName_MP"; showVar "Simulink:masks:GenSFuncShowModuleList_MP"; sfcnParam1 "Ts:"
      mask help: Simulink:masks:GenSFuncDesc_MD
      mask init: same as empirical_cell_twaice_balancing/Cell 1/ETA Model 1/ETA Model _sfcn
      settings: SFcnIsStateOwnerBlock=on
      settings: CopyFcn=|
      | if ~strcmp(get_param(gcb,'Linkstatus'),'none') && ...
      | ~strcmp(get_param(gcb,'Linkstatus'),'implicit')
      |   set_param(gcb,'LinkStatus','none');
      | end
      mask Help: eval('feval(''rtwprivate'',''rtwhelpview'',''rtw_sfcn_block'')');
      mask Display:
      | port_label('input',1,'SOC_init');
      | port_label('input',2,'T_init');
      | port_label('input',3,'I [A]');
      | port_label('input',4,'SOHc');
      | port_label('input',5,'Tcell');
      | port_label('output',1,'SOC');
  __InputSSForSFun__ : Subsystem
  __OutputSSForSFun__ : Subsystem
  SOC : Outport  VectorParamsAs1DForOutWhenUnconnected=off
  wires:
  SOC_init/1 -> __InputSSForSFun__/1(SOC_init)
  T_init/1 -> __InputSSForSFun__/2(T_init)
  I [A]/1 -> __InputSSForSFun__/3(I [A])
  SOHc/1 -> __InputSSForSFun__/4(SOHc)
  Tcell/1 -> __InputSSForSFun__/5(Tcell)
  __InputSSForSFun__/1(__UniqueOutportName__1__) -> SOC coloumb counting_sfcn/1
  __InputSSForSFun__/2(__UniqueOutportName__2__) -> SOC coloumb counting_sfcn/2
  __InputSSForSFun__/3(__UniqueOutportName__3__) -> SOC coloumb counting_sfcn/3
  __InputSSForSFun__/4(__UniqueOutportName__4__) -> SOC coloumb counting_sfcn/4
  __InputSSForSFun__/5(__UniqueOutportName__5__) -> SOC coloumb counting_sfcn/5
  SOC coloumb counting_sfcn/1 -> __OutputSSForSFun__/1(__UniqueInportName__1__)
  __OutputSSForSFun__/1(SOC) -> SOC/1

== system empirical_cell_twaice_balancing/Cell 4/ETA Model 1 ==
  "Current " : Inport  OutDataTypeStr=double  PortDimensions=1
  T_ambient / °C : Inport  Port=2  OutDataTypeStr=double  PortDimensions=1
  SOHc_init : Inport  Port=3
  SOHr_init : Inport  Port=4
  SOC_init : Inport  Port=5
  T_init : Inport  Port=6
  SOC_in : Inport  Port=7
  SOH : Inport  Port=8
  ETA Model _sfcn : S-Function  FunctionName=ETA_sf  Parameters=sfcnParam1, sfcnParam2, sfcnParam3  SFunctionModules=""  SFunctionDeploymentMode=off  EnableBusSupport=off  SFcnStateName=DWORK0,DWORK1,DWORK2,DWORK3,DWORK4,DWORK5,DWORK6,DWORK7,DWORK8,DWORK9,DWORK10,DWORK11,DWORK12,DWORK13,DWORK14,DWORK15,DWORK16,DWORK17,DWORK18,DWORK19,DWORK20,DWORK22,DWORK23,DWORK24,DWORK25,DWORK26,DWORK27,DWORK28,DWORK29,DWORK30,DWORK31,DWORK32,DWORK33,DWORK34,DWORK35,DWORK36  mask{rtw_sf_name=ETA_sf, showVar=off, sfcnParam1=sfcnParam1, sfcnParam2=sfcnParam2, sfcnParam3=sfcnParam3}
      mask prompts: rtw_sf_name "Simulink:masks:GenSFuncName_MP"; showVar "Simulink:masks:GenSFuncShowModuleList_MP"; sfcnParam1 "Ts:"; sfcnParam2 "act:"; sfcnParam3 "lic_no:"
      mask help: Simulink:masks:GenSFuncDesc_MD
      mask init: same as empirical_cell_twaice_balancing/Cell 1/ETA Model 1/ETA Model _sfcn
      settings: SFcnIsStateOwnerBlock=on
      settings: CopyFcn=|
      | if ~strcmp(get_param(gcb,'Linkstatus'),'none') && ...
      | ~strcmp(get_param(gcb,'Linkstatus'),'implicit')
      |   set_param(gcb,'LinkStatus','none');
      | end
      mask Help: eval('feval(''rtwprivate'',''rtwhelpview'',''rtw_sfcn_block'')');
      mask Display:
      | port_label('input',1,'Current ');
      | port_label('input',2,'T_ambient / °C');
      | port_label('input',3,'htc_in');
      | port_label('input',4,'Pcool_in');
      | port_label('input',5,'SOHc_init');
      | port_label('input',6,'SOHr_init');
      | port_label('input',7,'SOC_init');
      | port_label('input',8,'T_init');
      | port_label('input',9,'SOC_in');
      | port_label('input',10,'SOHc');
      | port_label('input',11,'SOHr');
      | port_label('output',1,'Current / A');
      | port_label('output',2,'Voltage / V');
      | port_label('output',3,'SOC / 0..1');
      | port_label('output',4,'SOHc / 0..1');
      | port_label('output',5,'T_sim / °C');
      | port_label('output',6,'Generated Heat / W');
      | port_label('output',7,'SOHr / 1');
      | port_label('output',8,'Power_sim / W');
      | port_label('output',9,'total_Ah');
  __InputSSForSFun__ : Subsystem
  __OutputSSForSFun__ : Subsystem
  Current / A : Outport  OutDataTypeStr=double  PortDimensions=1
  Voltage / V : Outport  Port=2  OutDataTypeStr=double  PortDimensions=1
  SOC / 0..1 : Outport  Port=3  OutDataTypeStr=double  PortDimensions=1
  SOHc / 0..1 : Outport  Port=4  OutDataTypeStr=double  PortDimensions=1
  T_sim / °C : Outport  Port=5  OutDataTypeStr=double  PortDimensions=1
  Generated Heat / W : Outport  Port=6  OutDataTypeStr=double  PortDimensions=1
  SOHr / 1 : Outport  Port=7  OutDataTypeStr=double  PortDimensions=1
  Power_sim / W : Outport  Port=8  OutDataTypeStr=double  PortDimensions=1
  total_Ah : Outport  Port=9
  wires:
  "Current "/1 -> __InputSSForSFun__/1("Current ")
  T_ambient / °C/1 -> __InputSSForSFun__/2(T_ambient / °C)
  SOHc_init/1 -> __InputSSForSFun__/3(SOHc_init)
  SOHr_init/1 -> __InputSSForSFun__/4(SOHr_init)
  SOC_init/1 -> __InputSSForSFun__/5(SOC_init)
  T_init/1 -> __InputSSForSFun__/6(T_init)
  SOC_in/1 -> __InputSSForSFun__/7(SOC_in)
  SOH/1 -> __InputSSForSFun__/8(SOH)
  __InputSSForSFun__/1(__UniqueOutportName__1__) -> ETA Model _sfcn/1
  __InputSSForSFun__/2(__UniqueOutportName__2__) -> ETA Model _sfcn/2
  __InputSSForSFun__/3(__UniqueOutportName__3__) -> ETA Model _sfcn/3
  __InputSSForSFun__/4(__UniqueOutportName__4__) -> ETA Model _sfcn/4
  __InputSSForSFun__/5(__UniqueOutportName__5__) -> ETA Model _sfcn/5
  __InputSSForSFun__/6(__UniqueOutportName__6__) -> ETA Model _sfcn/6
  __InputSSForSFun__/7(__UniqueOutportName__7__) -> ETA Model _sfcn/7
  __InputSSForSFun__/8(__UniqueOutportName__8__) -> ETA Model _sfcn/8
  __InputSSForSFun__/9(__UniqueOutportName__9__) -> ETA Model _sfcn/9
  __InputSSForSFun__/10(__UniqueOutportName__10__) -> ETA Model _sfcn/10
  __InputSSForSFun__/11(__UniqueOutportName__11__) -> ETA Model _sfcn/11
  ETA Model _sfcn/1 -> __OutputSSForSFun__/1(__UniqueInportName__1__)
  ETA Model _sfcn/2 -> __OutputSSForSFun__/2(__UniqueInportName__2__)
  ETA Model _sfcn/3 -> __OutputSSForSFun__/3(__UniqueInportName__3__)
  ETA Model _sfcn/4 -> __OutputSSForSFun__/4(__UniqueInportName__4__)
  ETA Model _sfcn/5 -> __OutputSSForSFun__/5(__UniqueInportName__5__)
  ETA Model _sfcn/6 -> __OutputSSForSFun__/6(__UniqueInportName__6__)
  ETA Model _sfcn/7 -> __OutputSSForSFun__/7(__UniqueInportName__7__)
  ETA Model _sfcn/8 -> __OutputSSForSFun__/8(__UniqueInportName__8__)
  ETA Model _sfcn/9 -> __OutputSSForSFun__/9(__UniqueInportName__9__)
  __OutputSSForSFun__/1(Current / A) -> Current / A/1
  __OutputSSForSFun__/2(Voltage / V) -> Voltage / V/1
  __OutputSSForSFun__/3(SOC / 0..1) -> SOC / 0..1/1
  __OutputSSForSFun__/4(SOHc / 0..1) -> SOHc / 0..1/1
  __OutputSSForSFun__/5(T_sim / °C) -> T_sim / °C/1
  __OutputSSForSFun__/6(Generated Heat / W) -> Generated Heat / W/1
  __OutputSSForSFun__/7(SOHr / 1) -> SOHr / 1/1
  __OutputSSForSFun__/8(Power_sim / W) -> Power_sim / W/1
  __OutputSSForSFun__/9(total_Ah) -> total_Ah/1

== system empirical_cell_twaice_balancing/Cell 4/SOC coloumb counting1 ==
  SOC_init : Inport
  T_init : Inport  Port=2
  I [A] : Inport  Port=3
  SOHc : Inport  Port=4
  Tcell : Inport  Port=5
  SOC coloumb counting_sfcn : S-Function  FunctionName=SOC_sf  Parameters=sfcnParam1  SFunctionModules=""  SFunctionDeploymentMode=off  EnableBusSupport=off  SFcnStateName=DWORK0,DWORK1  mask{rtw_sf_name=SOC_sf, showVar=off, sfcnParam1=sfcnParam1}
      mask prompts: rtw_sf_name "Simulink:masks:GenSFuncName_MP"; showVar "Simulink:masks:GenSFuncShowModuleList_MP"; sfcnParam1 "Ts:"
      mask help: Simulink:masks:GenSFuncDesc_MD
      mask init: same as empirical_cell_twaice_balancing/Cell 1/ETA Model 1/ETA Model _sfcn
      settings: SFcnIsStateOwnerBlock=on
      settings: CopyFcn=|
      | if ~strcmp(get_param(gcb,'Linkstatus'),'none') && ...
      | ~strcmp(get_param(gcb,'Linkstatus'),'implicit')
      |   set_param(gcb,'LinkStatus','none');
      | end
      mask Help: eval('feval(''rtwprivate'',''rtwhelpview'',''rtw_sfcn_block'')');
      mask Display:
      | port_label('input',1,'SOC_init');
      | port_label('input',2,'T_init');
      | port_label('input',3,'I [A]');
      | port_label('input',4,'SOHc');
      | port_label('input',5,'Tcell');
      | port_label('output',1,'SOC');
  __InputSSForSFun__ : Subsystem
  __OutputSSForSFun__ : Subsystem
  SOC : Outport  VectorParamsAs1DForOutWhenUnconnected=off
  wires:
  SOC_init/1 -> __InputSSForSFun__/1(SOC_init)
  T_init/1 -> __InputSSForSFun__/2(T_init)
  I [A]/1 -> __InputSSForSFun__/3(I [A])
  SOHc/1 -> __InputSSForSFun__/4(SOHc)
  Tcell/1 -> __InputSSForSFun__/5(Tcell)
  __InputSSForSFun__/1(__UniqueOutportName__1__) -> SOC coloumb counting_sfcn/1
  __InputSSForSFun__/2(__UniqueOutportName__2__) -> SOC coloumb counting_sfcn/2
  __InputSSForSFun__/3(__UniqueOutportName__3__) -> SOC coloumb counting_sfcn/3
  __InputSSForSFun__/4(__UniqueOutportName__4__) -> SOC coloumb counting_sfcn/4
  __InputSSForSFun__/5(__UniqueOutportName__5__) -> SOC coloumb counting_sfcn/5
  SOC coloumb counting_sfcn/1 -> __OutputSSForSFun__/1(__UniqueInportName__1__)
  __OutputSSForSFun__/1(SOC) -> SOC/1
